simulink model "dk"  (R2022b)
settings: Solver=VariableStepAuto  StartTime=0.0  StopTime=100  RelTol=1e-3
values from neighbouring files (symbols this model uses):
  A = J.A    [DK_iteration.m]    (also in Hinf_controller_hinfsyn.m = Jo.A; Hinf_controller_mixsyn.m = Jo.A; LQG_no_actuators.m)
  B = J.B    [DK_iteration.m]    (also in Hinf_controller_hinfsyn.m = Jo.B; Hinf_controller_mixsyn.m = Jo.B; LQG_no_actuators.m)
  C = J.C    [DK_iteration.m]    (also in Hinf_controller_hinfsyn.m = Jo.C; Hinf_controller_mixsyn.m = Jo.C; LQG_no_actuators.m)
  D = J.D    [DK_iteration.m]    (also in Hinf_controller_hinfsyn.m = Jo.D; Hinf_controller_mixsyn.m = Jo.D; LQG_no_actuators.m)
undefined symbols (not defined in the file or in its folder): A_DK, B_DK, C_DK, D_DK, X_start_mu
settings Model: Creator=alexi  LastModifiedBy=Giorgia

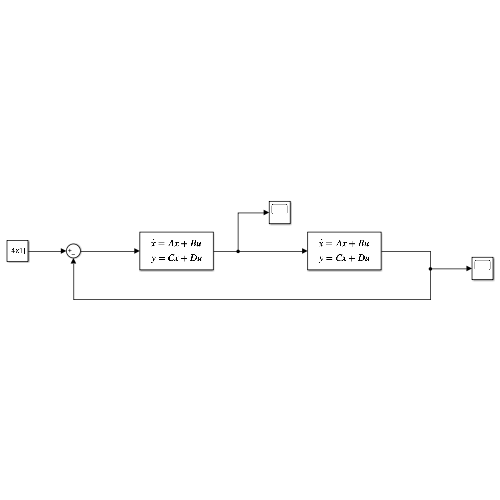
[thumbnail: Simulink's stored preview of the top-level diagram]
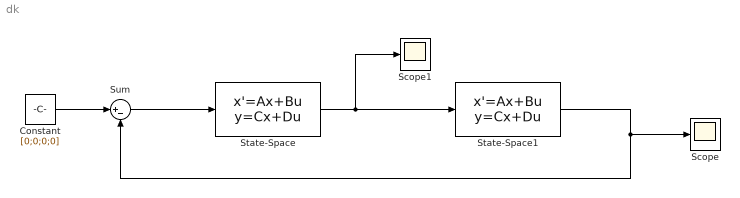
== system dk ==
  Constant : Constant  Value=[0;0;0;0]
  Scope : Scope
  Scope1 : Scope
  State-Space : StateSpace  A=A_DK  B=B_DK  C=C_DK  D=D_DK  InitialCondition=0
  State-Space1 : StateSpace  A=A  B=B  C=C  D=D  InitialCondition=X_start_mu
  Sum : Sum  Inputs=|+-
  wires:
  State-Space/1 -> State-Space1/1, Scope1/1
  Constant/1 -> Sum/1
  Sum/1 -> State-Space/1
  State-Space1/1 -> Scope/1, Sum/2
